simulink library "lib_converters"  (R2020b)
settings: Solver=VariableStepAuto  StartTime=0.0  StopTime=10.0  RelTol=1e-3
undefined symbols (not defined in the file): C_sc, DiscIntNeverNeededParam
libraries: powerlib x170, simulink x12, $bdroot x6, powerlib_meascontrol x3
(part 2 of 3)

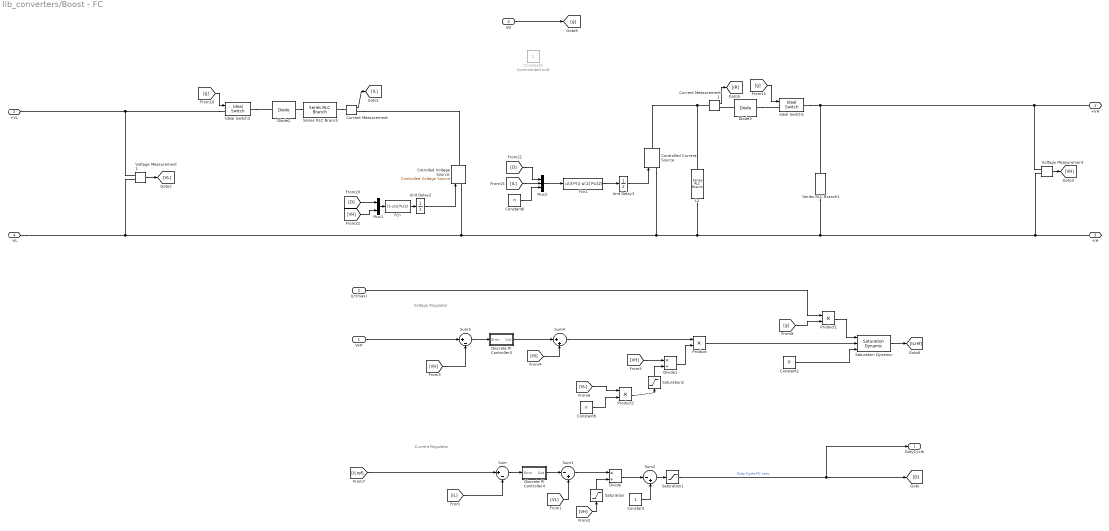
== system lib_converters/Boost - FC ==
  note: Current Regulator
  note: Voltage Regulator
  VH* : Inport
  IL*(max) : Inport  Port=2
  I/O : Inport  Port=3
  Constant : Constant
  Constant1 : Constant  Value=0
  Constant3 : Constant  Commented=on
  Constant6 : Constant  Value=n
  Constant8 : Constant  Value=n
  Controlled Current Source : powerlib/Electrical Sources/Controlled Current Source  Initialize=off  Source_Type=DC  Amplitude=0  Phase=0  Frequency=0  Measurements=None
  Cotrolled Voltage Source : powerlib/Electrical Sources/Controlled Voltage Source  Initialize=off  Source_Type=DC  Amplitude=0  Phase=0  Frequency=0  Measurements=None
  Current Measurement : powerlib/Measurements/Current Measurement  PhasorSimulation=off  OutputType=Complex  PSBequivalent=0
  Current Measurement1 : powerlib/Measurements/Current Measurement  PhasorSimulation=off  OutputType=Complex  PSBequivalent=0
  Diode2 : powerlib/Power Electronics/Diode  Ron=0.001  Lon=0  Vf=0  IC=0  UseSnubber=off  Rs=1e6  Cs=250e-9  Measurements=off
  Diode3 : powerlib/Power Electronics/Diode  Ron=0.001  Lon=0  Vf=0  IC=0  UseSnubber=off  Rs=1e6  Cs=250e-9  Measurements=off
  Discrete PI Controller3 : Subsystem  DialogController=POWERSYS.PowerSysDialog  mask(Discrete PI Controller){Kp=Kpv, Ki=Kiv, Par_Limits=[0.5 -0.5], Init=0, Ts=Tr}
      mask prompts: Kp "Proportional gain (Kp):"; Ki "Integral gain (Ki):"; Par_Limits "Output limits: [ Upper   Lower ]"; Init "Output initial value:"; Ts "Sample time:"
      mask help: This block implements a discrete PI controller.
      mask init:
      | UpperLimit=Par_Limits(1);
      | LowerLimit=Par_Limits(2);
      | power_initmask();
      mask Help: This block is part of a subset of blocks in the Extras library that does not have documentation associated with it, other than the block mask description.
      mask Display: disp('PI');
  Discrete PI Controller4 : Subsystem  DialogController=POWERSYS.PowerSysDialog  mask(Discrete PI Controller){Kp=Kpi/1000, Ki=Kii/1000, Par_Limits=[50 -50], Init=0, Ts=Ts}
      mask prompts: Kp "Proportional gain (Kp):"; Ki "Integral gain (Ki):"; Par_Limits "Output limits: [ Upper   Lower ]"; Init "Output initial value:"; Ts "Sample time:"
      mask help: This block implements a discrete PI controller.
      mask init:
      | UpperLimit=Par_Limits(1);
      | LowerLimit=Par_Limits(2);
      | power_initmask();
      mask Help: This block is part of a subset of blocks in the Extras library that does not have documentation associated with it, other than the block mask description.
      mask Display: disp('PI');
  Divide : Product  Inputs=*/  SampleTime=Ts
  Divide1 : Product  Inputs=*/  SampleTime=Ts
  Fcn : Fcn  Expr=(1-u(1))*u(2)
  Fcn1 : Fcn  Expr=u(3)*(1-u(1))*u(2)
  Ideal Switch1 : powerlib/Power Electronics/Ideal Switch  Ron=0.001  Lon=0  IC=0  Rs=1e5  Cs=inf  Measurements=off
  Ideal Switch3 : powerlib/Power Electronics/Ideal Switch  Ron=0.001  Lon=0  IC=0  Rs=1e5  Cs=inf  Measurements=off
  L2 : powerlib/Elements/Series RLC Branch  LConnTagsString=__new0  RConnTagsString=__new0  BranchType=C  Resistance=0.01  Inductance=100e-6  SetiL0=off  InitialCurrent=100  Capacitance=Co  Setx0=off  InitialVoltage=100  Measurements=None
  Mux1 : Mux  Inputs=2
  Mux2 : Mux  Inputs=3
  Product : Product  RndMeth=Zero
  Product1 : Product  RndMeth=Zero
  Product2 : Product  RndMeth=Zero
  Saturation : Saturate  UpperLimit=inf  LowerLimit=0.01  SampleTime=Ts
  Saturation Dynamic : simulink/Discontinuities/Saturation Dynamic  OutMin=[]  OutMax=[]  OutDataTypeStr=Inherit: Same as second input  OutDataType=fixdt(1, 16)  OutScaling=2^-10  DoSatur=off
  Saturation1 : Saturate  UpperLimit=1  LowerLimit=0  SampleTime=Ts
  Saturation2 : Saturate  UpperLimit=inf  LowerLimit=0.01  SampleTime=Ts
  Series RLC Branch : powerlib/Elements/Series RLC Branch  LConnTagsString=__new0  RConnTagsString=__new0  BranchType=L  Resistance=1  Inductance=L  SetiL0=off  InitialCurrent=1  Capacitance=1e-6  Setx0=off  InitialVoltage=0  Measurements=None
  Series RLC Branch1 : powerlib/Elements/Series RLC Branch  LConnTagsString=__new0  RConnTagsString=__new0  BranchType=R  Resistance=5e3  Inductance=1e-3  SetiL0=off  InitialCurrent=0  Capacitance=15  Setx0=on  InitialVoltage=270  Measurements=None
  Sum : Sum  Inputs=|+-
  Sum1 : Sum  Inputs=|-+
  Sum2 : Sum  Inputs=|-+
  Sum3 : Sum  Inputs=|+-
  Sum4 : Sum  Inputs=|++
  Unit Delay2 : UnitDelay  SampleTime=Ts  HasFrameUpgradeWarning=on
  Unit Delay3 : UnitDelay  SampleTime=Ts  HasFrameUpgradeWarning=on
  Voltage Measurement : powerlib/Measurements/Voltage Measurement  PhasorSimulation=off  OutputType=Complex  PSBequivalent=0
  Voltage Measurement1 : powerlib/Measurements/Voltage Measurement  PhasorSimulation=off  OutputType=Complex  PSBequivalent=0
  +VH : PMIOPort  Side=Right
  +VL : PMIOPort  Port=2  Side=Left
  -VH : PMIOPort  Port=3  Side=Right
  -VL : PMIOPort  Port=4  Side=Left
  DutyCycle : Outport
  wires:
  Product2/1 -> Saturation2/1
  Saturation1/1 -> [D], DutyCycle/1  "Duty Cycle FC conv"
  [IL] -> Mux2/2
  Sum3/1 -> Discrete PI Controller3/1(Error)
  [VH] -> Mux1/2
  Unit Delay3/1 -> Controlled Current Source/1
  Voltage Measurement/1 -> [VH]
  Discrete PI Controller3/1(Out) -> Sum4/1
  [D] -> Mux2/1
  Fcn1/1 -> Unit Delay3/1
  Fcn/1 -> Unit Delay2/1
  [D] -> Mux1/1
  Divide/1 -> Sum2/1
  Mux2/1 -> Fcn1/1
  Sum4/1 -> Product/1
  Constant8/1 -> Product2/2
  Constant6/1 -> Mux2/3
  IL*(max)/1 -> Product1/1
  Voltage Measurement1/1 -> [VL]
  Sum2/1 -> Saturation1/1
  Current Measurement1/1 -> [IR]
  [VH] -> Saturation/1
  Discrete PI Controller4/1(Out) -> Sum1/1
  [IL] -> Sum/2
  Sum/1 -> Discrete PI Controller4/1(Error)
  Product/1 -> Saturation Dynamic/2
  Constant/1 -> Sum2/2
  [VL] -> Product2/1
  Current Measurement/1 -> [IL]
  [VH] -> Sum3/2
  [VH] -> Divide1/1
  VH*/1 -> Sum3/1
  [IR] -> Sum4/2
  Mux1/1 -> Fcn/1
  Saturation/1 -> Divide/2
  Sum1/1 -> Divide/1
  [VL] -> Sum1/2
  Divide1/1 -> Product/2
  [ILref] -> Sum/1
  Constant1/1 -> Saturation Dynamic/3
  Saturation Dynamic/1 -> [ILref]
  [g] -> Ideal Switch3/1
  [g] -> Ideal Switch1/1
  Saturation2/1 -> Divide1/2
  [g] -> Product1/2
  Product1/1 -> Saturation Dynamic/1
  Unit Delay2/1 -> Cotrolled Voltage Source/1
  I/O/1 -> [g]
  connections:
  L2/LConn1 -- Controlled Current Source/RConn1 -- Current Measurement1/LConn1
  Ideal Switch3/LConn1 -- Voltage Measurement1/LConn1 -- +VL/RConn1
  Controlled Current Source/LConn1 -- L2/RConn1 -- -VH/RConn1 -- Voltage Measurement/LConn2 -- Series RLC Branch1/RConn1 -- Cotrolled Voltage Source/LConn1 -- Voltage Measurement1/LConn2 -- -VL/RConn1
  +VH/RConn1 -- Voltage Measurement/LConn1 -- Ideal Switch1/RConn1 -- Series RLC Branch1/LConn1
  Ideal Switch3/RConn1 -- Diode2/LConn1
  Diode2/RConn1 -- Series RLC Branch/LConn1
  Series RLC Branch/RConn1 -- Current Measurement/LConn1
  Current Measurement/RConn1 -- Cotrolled Voltage Source/RConn1
  Diode3/LConn1 -- Current Measurement1/RConn1
  Diode3/RConn1 -- Ideal Switch1/LConn1

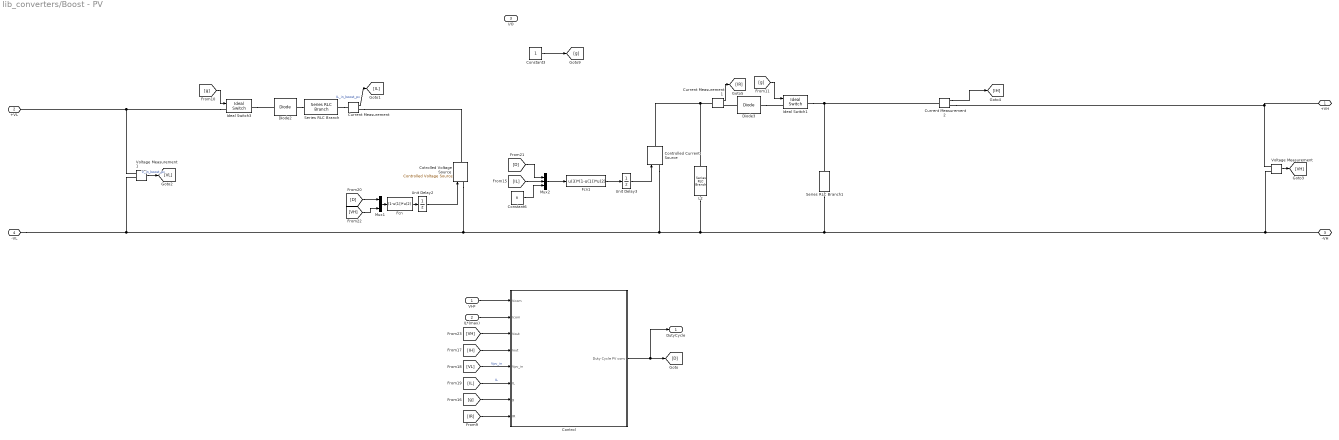
== system lib_converters/Boost - PV ==
  VH* : Inport
  IL*(max) : Inport  Port=2
  I/O : Inport  Port=3
  Constant3 : Constant
  Constant6 : Constant  Value=n
  Control : Subsystem  Variant=on  VariantControlMode=label  VariantControl=Choice  LabelModeActiveChoice=MPPT
  Controlled Current Source : powerlib/Electrical Sources/Controlled Current Source  Initialize=off  Source_Type=DC  Amplitude=0  Phase=0  Frequency=0  Measurements=None
  Cotrolled Voltage Source : powerlib/Electrical Sources/Controlled Voltage Source  Initialize=off  Source_Type=DC  Amplitude=0  Phase=0  Frequency=0  Measurements=None
  Current Measurement : powerlib/Measurements/Current Measurement  PhasorSimulation=off  OutputType=Complex  PSBequivalent=0
  Current Measurement1 : powerlib/Measurements/Current Measurement  PhasorSimulation=off  OutputType=Complex  PSBequivalent=0
  Current Measurement2 : powerlib/Measurements/Current Measurement  PhasorSimulation=off  OutputType=Complex  PSBequivalent=0
  Diode2 : powerlib/Power Electronics/Diode  Ron=0.001  Lon=0  Vf=0  IC=0  UseSnubber=off  Rs=1e6  Cs=250e-9  Measurements=off
  Diode3 : powerlib/Power Electronics/Diode  Ron=0.001  Lon=0  Vf=0  IC=0  UseSnubber=off  Rs=1e6  Cs=250e-9  Measurements=off
  Fcn : Fcn  Expr=(1-u(1))*u(2)
  Fcn1 : Fcn  Expr=u(3)*(1-u(1))*u(2)
  Ideal Switch1 : powerlib/Power Electronics/Ideal Switch  Ron=0.001  Lon=0  IC=0  Rs=1e5  Cs=inf  Measurements=off
  Ideal Switch3 : powerlib/Power Electronics/Ideal Switch  Ron=0.001  Lon=0  IC=0  Rs=1e5  Cs=inf  Measurements=off
  L2 : powerlib/Elements/Series RLC Branch  LConnTagsString=__new0  RConnTagsString=__new0  BranchType=C  Resistance=0.01  Inductance=100e-6  SetiL0=off  InitialCurrent=100  Capacitance=Co  Setx0=off  InitialVoltage=100  Measurements=None
  Mux1 : Mux  Inputs=2
  Mux2 : Mux  Inputs=3
  Series RLC Branch : powerlib/Elements/Series RLC Branch  LConnTagsString=__new0  RConnTagsString=__new0  BranchType=L  Resistance=1  Inductance=L  SetiL0=off  InitialCurrent=1  Capacitance=1e-6  Setx0=off  InitialVoltage=0  Measurements=None
  Series RLC Branch1 : powerlib/Elements/Series RLC Branch  LConnTagsString=__new0  RConnTagsString=__new0  BranchType=R  Resistance=5e3  Inductance=1e-3  SetiL0=off  InitialCurrent=0  Capacitance=15  Setx0=on  InitialVoltage=270  Measurements=None
  Unit Delay2 : UnitDelay  SampleTime=Ts  HasFrameUpgradeWarning=on
  Unit Delay3 : UnitDelay  SampleTime=Ts  HasFrameUpgradeWarning=on
  Voltage Measurement : powerlib/Measurements/Voltage Measurement  PhasorSimulation=off  OutputType=Complex  PSBequivalent=0
  Voltage Measurement1 : powerlib/Measurements/Voltage Measurement  PhasorSimulation=off  OutputType=Complex  PSBequivalent=0
  +VH : PMIOPort  Side=Right
  +VL : PMIOPort  Port=2  Side=Left
  -VH : PMIOPort  Port=3  Side=Right
  -VL : PMIOPort  Port=4  Side=Left
  DutyCycle : Outport
  wires:
  Constant3/1 -> [g]
  [IL] -> Mux2/2
  [VH] -> Mux1/2
  Unit Delay3/1 -> Controlled Current Source/1
  Voltage Measurement/1 -> [VH]
  [D] -> Mux2/1
  Fcn1/1 -> Unit Delay3/1
  Fcn/1 -> Unit Delay2/1
  [D] -> Mux1/1
  Mux2/1 -> Fcn1/1
  Constant6/1 -> Mux2/3
  IL*(max)/1 -> Control/2(Icom)
  Voltage Measurement1/1 -> [VL]  "V_in_boost_pv"
  Current Measurement1/1 -> [IR]
  Current Measurement/1 -> [IL]  "IL_in_boost_pv"
  VH*/1 -> Control/1(Vcom)
  Mux1/1 -> Fcn/1
  [g] -> Ideal Switch3/1
  [g] -> Ideal Switch1/1
  Unit Delay2/1 -> Cotrolled Voltage Source/1
  Current Measurement2/1 -> [IH]
  [VH] -> Control/3(Vout)
  [IH] -> Control/4(Iout)
  [VL] -> Control/5(Vpv_in)  "Vpv_in"
  [IL] -> Control/6(IL)  "IL"
  [g] -> Control/7(g)
  [IR] -> Control/8(IR)
  Control/1(Duty Cycle PV conv) -> DutyCycle/1, [D]
  connections:
  L2/LConn1 -- Controlled Current Source/RConn1 -- Current Measurement1/LConn1
  Ideal Switch3/LConn1 -- Voltage Measurement1/LConn1 -- +VL/RConn1
  Controlled Current Source/LConn1 -- L2/RConn1 -- -VH/RConn1 -- Voltage Measurement/LConn2 -- Series RLC Branch1/RConn1 -- Cotrolled Voltage Source/LConn1 -- Voltage Measurement1/LConn2 -- -VL/RConn1
  +VH/RConn1 -- Current Measurement2/RConn1 -- Voltage Measurement/LConn1
  Ideal Switch3/RConn1 -- Diode2/LConn1
  Diode2/RConn1 -- Series RLC Branch/LConn1
  Series RLC Branch/RConn1 -- Current Measurement/LConn1
  Current Measurement/RConn1 -- Cotrolled Voltage Source/RConn1
  Diode3/LConn1 -- Current Measurement1/RConn1
  Diode3/RConn1 -- Ideal Switch1/LConn1
  Ideal Switch1/RConn1 -- Current Measurement2/LConn1 -- Series RLC Branch1/LConn1

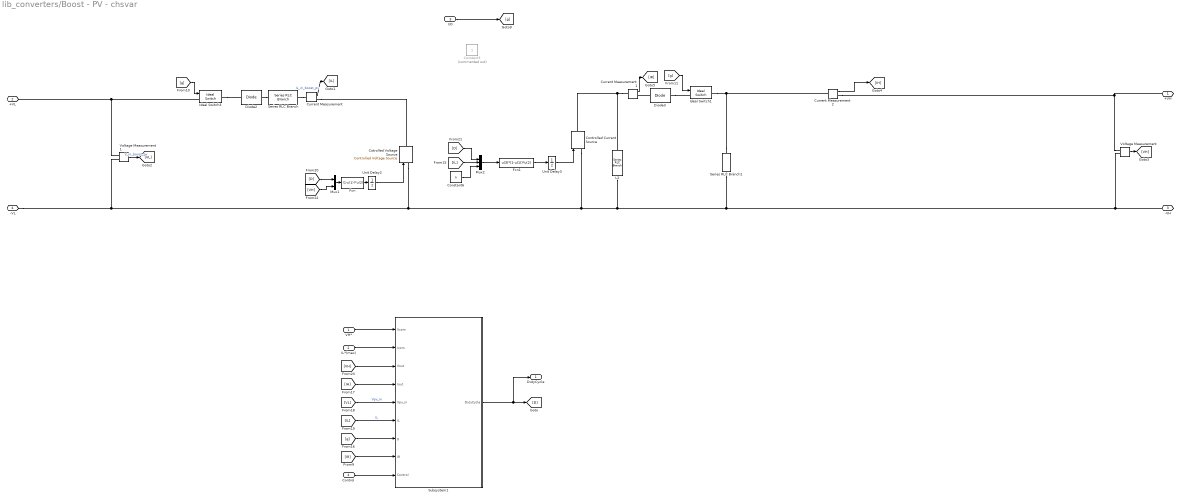
== system lib_converters/Boost - PV - chsvar ==
  VH* : Inport
  IL*(max) : Inport  Port=2
  I/O : Inport  Port=3
  Control : Inport  Port=4
  Constant3 : Constant  Commented=on
  Constant6 : Constant  Value=n
  Controlled Current Source : powerlib/Electrical Sources/Controlled Current Source  Initialize=off  Source_Type=DC  Amplitude=0  Phase=0  Frequency=0  Measurements=None
  Cotrolled Voltage Source : powerlib/Electrical Sources/Controlled Voltage Source  Initialize=off  Source_Type=DC  Amplitude=0  Phase=0  Frequency=0  Measurements=None
  Current Measurement : powerlib/Measurements/Current Measurement  PhasorSimulation=off  OutputType=Complex  PSBequivalent=0
  Current Measurement1 : powerlib/Measurements/Current Measurement  PhasorSimulation=off  OutputType=Complex  PSBequivalent=0
  Current Measurement2 : powerlib/Measurements/Current Measurement  PhasorSimulation=off  OutputType=Complex  PSBequivalent=0
  Diode2 : powerlib/Power Electronics/Diode  Ron=0.001  Lon=0  Vf=0  IC=0  UseSnubber=off  Rs=1e6  Cs=250e-9  Measurements=off
  Diode3 : powerlib/Power Electronics/Diode  Ron=0.001  Lon=0  Vf=0  IC=0  UseSnubber=off  Rs=1e6  Cs=250e-9  Measurements=off
  Fcn : Fcn  Expr=(1-u(1))*u(2)
  Fcn1 : Fcn  Expr=u(3)*(1-u(1))*u(2)
  Ideal Switch1 : powerlib/Power Electronics/Ideal Switch  Ron=0.001  Lon=0  IC=0  Rs=1e5  Cs=inf  Measurements=off
  Ideal Switch3 : powerlib/Power Electronics/Ideal Switch  Ron=0.001  Lon=0  IC=0  Rs=1e5  Cs=inf  Measurements=off
  L2 : powerlib/Elements/Series RLC Branch  LConnTagsString=__new0  RConnTagsString=__new0  BranchType=C  Resistance=0.01  Inductance=100e-6  SetiL0=off  InitialCurrent=100  Capacitance=Co  Setx0=off  InitialVoltage=100  Measurements=None
  Mux1 : Mux  Inputs=2
  Mux2 : Mux  Inputs=3
  Series RLC Branch : powerlib/Elements/Series RLC Branch  LConnTagsString=__new0  RConnTagsString=__new0  BranchType=L  Resistance=1  Inductance=L  SetiL0=off  InitialCurrent=1  Capacitance=1e-6  Setx0=off  InitialVoltage=0  Measurements=None
  Series RLC Branch1 : powerlib/Elements/Series RLC Branch  LConnTagsString=__new0  RConnTagsString=__new0  BranchType=R  Resistance=5e3  Inductance=1e-3  SetiL0=off  InitialCurrent=0  Capacitance=15  Setx0=on  InitialVoltage=270  Measurements=None
  Subsystem1 : Subsystem
  Unit Delay2 : UnitDelay  SampleTime=Ts  HasFrameUpgradeWarning=on
  Unit Delay3 : UnitDelay  SampleTime=Ts  HasFrameUpgradeWarning=on
  Voltage Measurement : powerlib/Measurements/Voltage Measurement  PhasorSimulation=off  OutputType=Complex  PSBequivalent=0
  Voltage Measurement1 : powerlib/Measurements/Voltage Measurement  PhasorSimulation=off  OutputType=Complex  PSBequivalent=0
  +VH : PMIOPort  Side=Right
  +VL : PMIOPort  Port=2  Side=Left
  -VH : PMIOPort  Port=3  Side=Right
  -VL : PMIOPort  Port=4  Side=Left
  DutyCycle : Outport
  wires:
  Subsystem1/1(DutyCycle) -> [D], DutyCycle/1
  [IR] -> Subsystem1/8(IR)
  [g] -> Subsystem1/7(g)
  [IL] -> Subsystem1/6(IL)  "IL"
  [VL] -> Subsystem1/5(Vpv_in)  "Vpv_in"
  [IH] -> Subsystem1/4(Iout)
  [VH] -> Subsystem1/3(Vout)
  Current Measurement2/1 -> [IH]
  Unit Delay2/1 -> Cotrolled Voltage Source/1
  [g] -> Ideal Switch1/1
  [g] -> Ideal Switch3/1
  Mux1/1 -> Fcn/1
  VH*/1 -> Subsystem1/1(Vcom)
  Current Measurement/1 -> [IL]  "IL_in_boost_pv"
  Current Measurement1/1 -> [IR]
  Voltage Measurement1/1 -> [VL]  "V_in_boost_pv"
  IL*(max)/1 -> Subsystem1/2(Icom)
  Constant6/1 -> Mux2/3
  Mux2/1 -> Fcn1/1
  [D] -> Mux1/1
  Fcn/1 -> Unit Delay2/1
  Fcn1/1 -> Unit Delay3/1
  [D] -> Mux2/1
  Voltage Measurement/1 -> [VH]
  Unit Delay3/1 -> Controlled Current Source/1
  [VH] -> Mux1/2
  [IL] -> Mux2/2
  Control/1 -> Subsystem1/9(Control)
  I/O/1 -> [g]
  connections:
  Series RLC Branch1/LConn1 -- Current Measurement2/LConn1 -- Ideal Switch1/RConn1
  Diode3/RConn1 -- Ideal Switch1/LConn1
  Diode3/LConn1 -- Current Measurement1/RConn1
  Current Measurement/RConn1 -- Cotrolled Voltage Source/RConn1
  Series RLC Branch/RConn1 -- Current Measurement/LConn1
  Diode2/RConn1 -- Series RLC Branch/LConn1
  Ideal Switch3/RConn1 -- Diode2/LConn1
  Voltage Measurement/LConn1 -- Current Measurement2/RConn1 -- +VH/RConn1
  -VL/RConn1 -- Voltage Measurement1/LConn2 -- Cotrolled Voltage Source/LConn1 -- Series RLC Branch1/RConn1 -- Voltage Measurement/LConn2 -- -VH/RConn1 -- L2/RConn1 -- Controlled Current Source/LConn1
  +VL/RConn1 -- Voltage Measurement1/LConn1 -- Ideal Switch3/LConn1
  Current Measurement1/LConn1 -- Controlled Current Source/RConn1 -- L2/LConn1

== system lib_converters/Boost - PV - fast ==
  I/O : Inport
  Constant6 : Constant  Value=n
  Controlled Current Source : powerlib/Electrical Sources/Controlled Current Source  Initialize=off  Source_Type=DC  Amplitude=0  Phase=0  Frequency=0  Measurements=None
  Cotrolled Voltage Source : powerlib/Electrical Sources/Controlled Voltage Source  Initialize=off  Source_Type=DC  Amplitude=0  Phase=0  Frequency=0  Measurements=None
  Current Measurement : powerlib/Measurements/Current Measurement  PhasorSimulation=off  OutputType=Complex  PSBequivalent=0
  Current Measurement1 : powerlib/Measurements/Current Measurement  PhasorSimulation=off  OutputType=Complex  PSBequivalent=0
  Current Measurement2 : powerlib/Measurements/Current Measurement  PhasorSimulation=off  OutputType=Complex  PSBequivalent=0
  Diode2 : powerlib/Power Electronics/Diode  Ron=0.001  Lon=0  Vf=0  IC=0  UseSnubber=off  Rs=1e6  Cs=250e-9  Measurements=off
  Diode3 : powerlib/Power Electronics/Diode  Ron=0.001  Lon=0  Vf=0  IC=0  UseSnubber=off  Rs=1e6  Cs=250e-9  Measurements=off
  Fcn : Fcn  Expr=(1-u(1))*u(2)
  Fcn1 : Fcn  Expr=u(3)*(1-u(1))*u(2)
  Ideal Switch1 : powerlib/Power Electronics/Ideal Switch  Ron=0.001  Lon=0  IC=0  Rs=1e5  Cs=inf  Measurements=off
  Ideal Switch3 : powerlib/Power Electronics/Ideal Switch  Ron=0.001  Lon=0  IC=0  Rs=1e5  Cs=inf  Measurements=off
  L2 : powerlib/Elements/Series RLC Branch  LConnTagsString=__new0  RConnTagsString=__new0  BranchType=C  Resistance=0.01  Inductance=100e-6  SetiL0=off  InitialCurrent=100  Capacitance=Co  Setx0=off  InitialVoltage=100  Measurements=None
  MPPT : MATLAB Function  TreatAsAtomicUnit=on
  Mux1 : Mux  Inputs=2
  Mux2 : Mux  Inputs=3
  Saturation1 : Saturate  UpperLimit=1  LowerLimit=0  SampleTime=Ts
  Series RLC Branch : powerlib/Elements/Series RLC Branch  LConnTagsString=__new0  RConnTagsString=__new0  BranchType=L  Resistance=1  Inductance=L  SetiL0=off  InitialCurrent=1  Capacitance=1e-6  Setx0=off  InitialVoltage=0  Measurements=None
  Series RLC Branch1 : powerlib/Elements/Series RLC Branch  LConnTagsString=__new0  RConnTagsString=__new0  BranchType=R  Resistance=5e3  Inductance=1e-3  SetiL0=off  InitialCurrent=0  Capacitance=15  Setx0=on  InitialVoltage=270  Measurements=None
  Unit Delay1 : UnitDelay  SampleTime=Ts*10  HasFrameUpgradeWarning=on
  Unit Delay2 : UnitDelay  SampleTime=Ts  HasFrameUpgradeWarning=on
  Unit Delay3 : UnitDelay  SampleTime=Ts  HasFrameUpgradeWarning=on
  Voltage Measurement : powerlib/Measurements/Voltage Measurement  PhasorSimulation=off  OutputType=Complex  PSBequivalent=0
  Voltage Measurement1 : powerlib/Measurements/Voltage Measurement  PhasorSimulation=off  OutputType=Complex  PSBequivalent=0
  +VH : PMIOPort  Side=Right
  +VL : PMIOPort  Port=2  Side=Left
  -VH : PMIOPort  Port=3  Side=Right
  -VL : PMIOPort  Port=4  Side=Left
  wires:
  [IL] -> MPPT/2(I_L)  "IL"
  [VL] -> MPPT/1(Vpv_in)  "Vpv_in"
  Current Measurement2/1 -> [IH]
  Unit Delay2/1 -> Cotrolled Voltage Source/1
  [g] -> Ideal Switch1/1
  [g] -> Ideal Switch3/1
  Mux1/1 -> Fcn/1
  Current Measurement/1 -> [IL]  "IL_in_boost_pv"
  Current Measurement1/1 -> [IR]
  Voltage Measurement1/1 -> [VL]  "V_in_boost_pv"
  Constant6/1 -> Mux2/3
  Mux2/1 -> Fcn1/1
  [D] -> Mux1/1
  Fcn/1 -> Unit Delay2/1
  Fcn1/1 -> Unit Delay3/1
  [D] -> Mux2/1
  Voltage Measurement/1 -> [VH]
  Unit Delay3/1 -> Controlled Current Source/1
  [VH] -> Mux1/2
  [IL] -> Mux2/2
  I/O/1 -> [g]
  Unit Delay1/1 -> Saturation1/1
  MPPT/1(D) -> Unit Delay1/1
  Saturation1/1 -> [D]  "Duty Cycle PV conv"
  connections:
  Series RLC Branch1/LConn1 -- Current Measurement2/LConn1 -- Ideal Switch1/RConn1
  Diode3/RConn1 -- Ideal Switch1/LConn1
  Diode3/LConn1 -- Current Measurement1/RConn1
  Current Measurement/RConn1 -- Cotrolled Voltage Source/RConn1
  Series RLC Branch/RConn1 -- Current Measurement/LConn1
  Diode2/RConn1 -- Series RLC Branch/LConn1
  Ideal Switch3/RConn1 -- Diode2/LConn1
  Voltage Measurement/LConn1 -- Current Measurement2/RConn1 -- +VH/RConn1
  -VL/RConn1 -- Voltage Measurement1/LConn2 -- Cotrolled Voltage Source/LConn1 -- Series RLC Branch1/RConn1 -- Voltage Measurement/LConn2 -- -VH/RConn1 -- L2/RConn1 -- Controlled Current Source/LConn1
  +VL/RConn1 -- Voltage Measurement1/LConn1 -- Ideal Switch3/LConn1
  Current Measurement1/LConn1 -- Controlled Current Source/RConn1 -- L2/LConn1

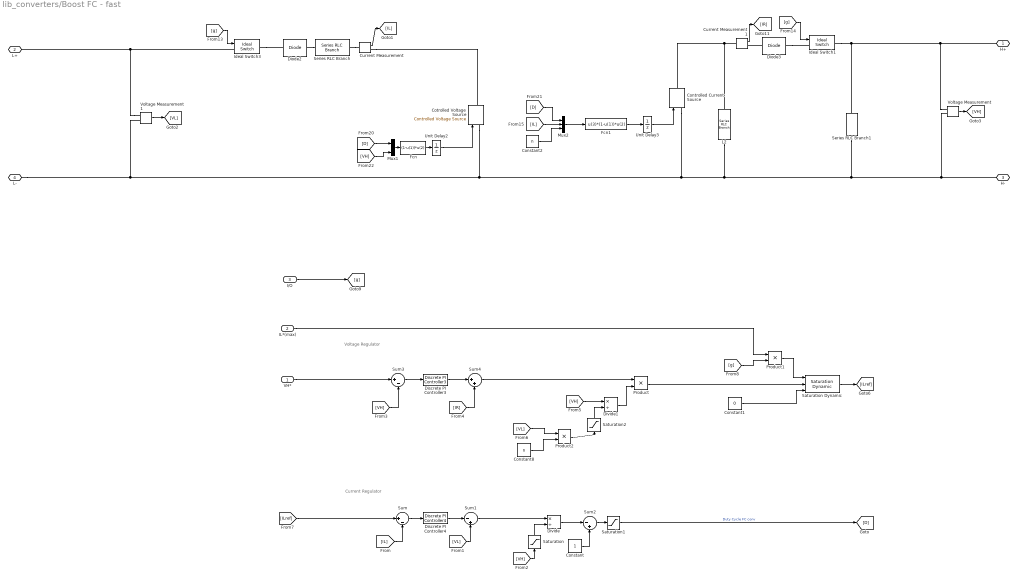
== system lib_converters/Boost FC - fast ==
  note: Voltage Regulator
  note: Current Regulator
  VH* : Inport
  IL*(max) : Inport  Port=2
  I/O : Inport  Port=3
  Constant : Constant
  Constant1 : Constant  Value=0
  Constant2 : Constant  Value=n
  Constant8 : Constant  Value=n
  Controlled Current Source : powerlib/Electrical Sources/Controlled Current Source  Initialize=off  Source_Type=DC  Amplitude=0  Phase=0  Frequency=0  Measurements=None
  Cotrolled Voltage Source : powerlib/Electrical Sources/Controlled Voltage Source  Initialize=off  Source_Type=DC  Amplitude=0  Phase=0  Frequency=0  Measurements=None
  Current Measurement : powerlib/Measurements/Current Measurement  PhasorSimulation=off  OutputType=Complex  PSBequivalent=0
  Current Measurement1 : powerlib/Measurements/Current Measurement  PhasorSimulation=off  OutputType=Complex  PSBequivalent=0
  Diode2 : powerlib/Power Electronics/Diode  Ron=0.001  Lon=0  Vf=0  IC=0  UseSnubber=off  Rs=1e6  Cs=250e-9  Measurements=off
  Diode3 : powerlib/Power Electronics/Diode  Ron=0.001  Lon=0  Vf=0  IC=0  UseSnubber=off  Rs=1e6  Cs=250e-9  Measurements=off
  Discrete PI Controller3 : $bdroot/Boost - FC/Discrete PI Controller3  Kp=Kpv  Ki=Kiv  Par_Limits=[0.5 -0.5]  Init=0  Ts=Ts
  Discrete PI Controller4 : $bdroot/Boost - FC/Discrete PI Controller4  Kp=Kpi/1000  Ki=Kii/1000  Par_Limits=[50 -50]  Init=0  Ts=Ts
  Divide : Product  Inputs=*/  SampleTime=Ts
  Divide1 : Product  Inputs=*/  SampleTime=Ts
  Fcn : Fcn  Expr=(1-u(1))*u(2)
  Fcn1 : Fcn  Expr=u(3)*(1-u(1))*u(2)
  Ideal Switch1 : powerlib/Power Electronics/Ideal Switch  Ron=0.001  Lon=0  IC=0  Rs=1e5  Cs=inf  Measurements=off
  Ideal Switch3 : powerlib/Power Electronics/Ideal Switch  Ron=0.001  Lon=0  IC=0  Rs=1e5  Cs=inf  Measurements=off
  L2 : powerlib/Elements/Series RLC Branch  LConnTagsString=__new0  RConnTagsString=__new0  BranchType=C  Resistance=0.01  Inductance=100e-6  SetiL0=off  InitialCurrent=100  Capacitance=Co  Setx0=off  InitialVoltage=100  Measurements=None
  Mux1 : Mux  Inputs=2
  Mux2 : Mux  Inputs=3
  Product : Product  RndMeth=Zero
  Product1 : Product  RndMeth=Zero
  Product2 : Product  RndMeth=Zero
  Saturation : Saturate  UpperLimit=inf  LowerLimit=0.01  SampleTime=Ts
  Saturation Dynamic : simulink/Discontinuities/Saturation Dynamic  OutMin=[]  OutMax=[]  OutDataTypeStr=Inherit: Same as second input  OutDataType=fixdt(1, 16)  OutScaling=2^-10  DoSatur=off
  Saturation1 : Saturate  UpperLimit=1  LowerLimit=0  SampleTime=Ts
  Saturation2 : Saturate  UpperLimit=inf  LowerLimit=0.01  SampleTime=Ts
  Series RLC Branch : powerlib/Elements/Series RLC Branch  LConnTagsString=__new0  RConnTagsString=__new0  BranchType=L  Resistance=1  Inductance=L  SetiL0=off  InitialCurrent=1  Capacitance=1e-6  Setx0=off  InitialVoltage=0  Measurements=None
  Series RLC Branch1 : powerlib/Elements/Series RLC Branch  LConnTagsString=__new0  RConnTagsString=__new0  BranchType=R  Resistance=5e3  Inductance=1e-3  SetiL0=off  InitialCurrent=0  Capacitance=15  Setx0=on  InitialVoltage=270  Measurements=None
  Sum : Sum  Inputs=|+-
  Sum1 : Sum  Inputs=|-+
  Sum2 : Sum  Inputs=|-+
  Sum3 : Sum  Inputs=|+-
  Sum4 : Sum  Inputs=|++
  Unit Delay2 : UnitDelay  SampleTime=Ts  HasFrameUpgradeWarning=on
  Unit Delay3 : UnitDelay  SampleTime=Ts  HasFrameUpgradeWarning=on
  Voltage Measurement : powerlib/Measurements/Voltage Measurement  PhasorSimulation=off  OutputType=Complex  PSBequivalent=0
  Voltage Measurement1 : powerlib/Measurements/Voltage Measurement  PhasorSimulation=off  OutputType=Complex  PSBequivalent=0
  H+ : PMIOPort  Side=Right
  L+ : PMIOPort  Port=2  Side=Left
  H- : PMIOPort  Port=3  Side=Right
  L- : PMIOPort  Port=4  Side=Left
  wires:
  IL*(max)/1 -> Product1/1
  Divide1/1 -> Product/2
  [ILref] -> Sum/1
  Sum1/1 -> Divide/1
  [VH] -> Divide1/1
  [VL] -> Sum1/2
  [IR] -> Sum4/2
  Constant/1 -> Sum2/2
  Product/1 -> Saturation Dynamic/2
  [IL] -> Sum/2
  Discrete PI Controller4/1 -> Sum1/1
  Divide/1 -> Sum2/1
  Saturation1/1 -> [D]  "Duty Cycle FC conv"
  Constant8/1 -> Product2/2
  Sum3/1 -> Discrete PI Controller3/1
  VH*/1 -> Sum3/1
  I/O/1 -> [g]
  Saturation2/1 -> Divide1/2
  Constant1/1 -> Saturation Dynamic/3
  Sum2/1 -> Saturation1/1
  [VL] -> Product2/1
  [g] -> Product1/2
  Saturation Dynamic/1 -> [ILref]
  Saturation/1 -> Divide/2
  [VH] -> Saturation/1
  Discrete PI Controller3/1 -> Sum4/1
  [VH] -> Sum3/2
  Product1/1 -> Saturation Dynamic/1
  Product2/1 -> Saturation2/1
  Sum4/1 -> Product/1
  Sum/1 -> Discrete PI Controller4/1
  [g] -> Ideal Switch1/1
  Voltage Measurement1/1 -> [VL]
  Current Measurement/1 -> [IL]
  Fcn/1 -> Unit Delay2/1
  [D] -> Mux2/1
  Unit Delay2/1 -> Cotrolled Voltage Source/1
  Mux1/1 -> Fcn/1
  Voltage Measurement/1 -> [VH]
  [VH] -> Mux1/2
  Current Measurement1/1 -> [IR]
  Mux2/1 -> Fcn1/1
  Unit Delay3/1 -> Controlled Current Source/1
  [D] -> Mux1/1
  Fcn1/1 -> Unit Delay3/1
  Constant2/1 -> Mux2/3
  [g] -> Ideal Switch3/1
  [IL] -> Mux2/2
  connections:
  Voltage Measurement/LConn1 -- H+/RConn1 -- Series RLC Branch1/LConn1 -- Ideal Switch1/RConn1
  Voltage Measurement/LConn2 -- Series RLC Branch1/RConn1 -- Controlled Current Source/LConn1 -- Cotrolled Voltage Source/LConn1 -- Voltage Measurement1/LConn2 -- L-/RConn1 -- L2/RConn1 -- H-/RConn1
  Controlled Current Source/RConn1 -- Current Measurement1/LConn1 -- L2/LConn1
  Voltage Measurement1/LConn1 -- L+/RConn1 -- Ideal Switch3/LConn1
  Diode3/LConn1 -- Current Measurement1/RConn1
  Ideal Switch3/RConn1 -- Diode2/LConn1
  Diode3/RConn1 -- Ideal Switch1/LConn1
  Series RLC Branch/RConn1 -- Current Measurement/LConn1
  Current Measurement/RConn1 -- Cotrolled Voltage Source/RConn1
  Diode2/RConn1 -- Series RLC Branch/LConn1

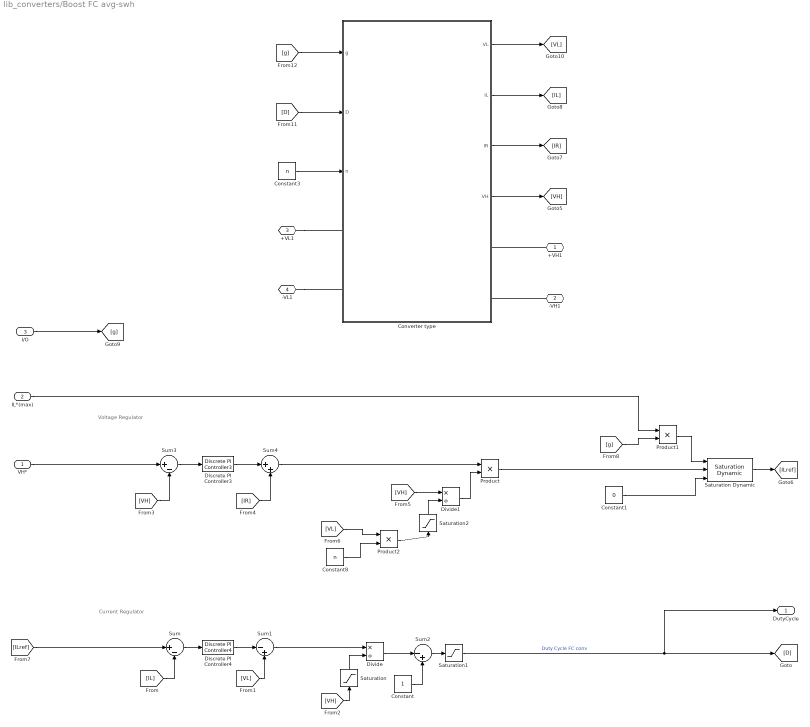
== system lib_converters/Boost FC avg-swh ==
  note: Voltage Regulator
  note: Current Regulator
  VH* : Inport
  IL*(max) : Inport  Port=2
  I/O : Inport  Port=3
  Constant : Constant
  Constant1 : Constant  Value=0
  Constant3 : Constant  Value=n
  Constant8 : Constant  Value=n
  Converter type : Subsystem  Variant=on  VariantControlMode=label  VariantControl=Choice  LabelModeActiveChoice=Choice
  Discrete PI Controller3 : $bdroot/Boost - FC/Discrete PI Controller3  Kp=Kpv  Ki=Kiv  Par_Limits=[0.5 -0.5]  Init=0  Ts=Ts
  Discrete PI Controller4 : $bdroot/Boost - FC/Discrete PI Controller4  Kp=Kpi/1000  Ki=Kii/1000  Par_Limits=[50 -50]  Init=0  Ts=Ts
  Divide : Product  Inputs=*/  SampleTime=Ts
  Divide1 : Product  Inputs=*/  SampleTime=Ts
  Product : Product  RndMeth=Zero
  Product1 : Product  RndMeth=Zero
  Product2 : Product  RndMeth=Zero
  Saturation : Saturate  UpperLimit=inf  LowerLimit=0.01  SampleTime=Ts
  Saturation Dynamic : simulink/Discontinuities/Saturation Dynamic  OutMin=[]  OutMax=[]  OutDataTypeStr=Inherit: Same as second input  OutDataType=fixdt(1, 16)  OutScaling=2^-10  DoSatur=off
  Saturation1 : Saturate  UpperLimit=1  LowerLimit=0  SampleTime=Ts
  Saturation2 : Saturate  UpperLimit=inf  LowerLimit=0.01  SampleTime=Ts
  Sum : Sum  Inputs=|+-
  Sum1 : Sum  Inputs=|-+
  Sum2 : Sum  Inputs=|-+
  Sum3 : Sum  Inputs=|+-
  Sum4 : Sum  Inputs=|++
  +VH1 : PMIOPort  Side=Right
  -VH1 : PMIOPort  Port=2  Side=Right
  +VL1 : PMIOPort  Port=3  Side=Left
  -VL1 : PMIOPort  Port=4  Side=Left
  DutyCycle : Outport
  wires:
  IL*(max)/1 -> Product1/1
  Divide1/1 -> Product/2
  [ILref] -> Sum/1
  Sum1/1 -> Divide/1
  [VH] -> Divide1/1
  [VL] -> Sum1/2
  [IR] -> Sum4/2
  Constant/1 -> Sum2/2
  Product/1 -> Saturation Dynamic/2
  [IL] -> Sum/2
  Discrete PI Controller4/1 -> Sum1/1
  Divide/1 -> Sum2/1
  Saturation1/1 -> [D], DutyCycle/1  "Duty Cycle FC conv"
  Constant8/1 -> Product2/2
  Sum3/1 -> Discrete PI Controller3/1
  VH*/1 -> Sum3/1
  I/O/1 -> [g]
  Saturation2/1 -> Divide1/2
  Constant1/1 -> Saturation Dynamic/3
  Sum2/1 -> Saturation1/1
  [VL] -> Product2/1
  [g] -> Product1/2
  Saturation Dynamic/1 -> [ILref]
  Saturation/1 -> Divide/2
  [VH] -> Saturation/1
  Discrete PI Controller3/1 -> Sum4/1
  [VH] -> Sum3/2
  Product1/1 -> Saturation Dynamic/1
  Product2/1 -> Saturation2/1
  Sum4/1 -> Product/1
  Sum/1 -> Discrete PI Controller4/1
  Converter type/4(VH) -> [VH]
  Converter type/3(IR) -> [IR]
  Converter type/2(IL) -> [IL]
  Converter type/1(VL) -> [VL]
  [g] -> Converter type/1(g)
  [D] -> Converter type/2(D)
  Constant3/1 -> Converter type/3(n)
  connections:
  -VH1/RConn1 -- Converter type/RConn2
  +VH1/RConn1 -- Converter type/RConn1
  +VL1/RConn1 -- Converter type/LConn1
  -VL1/RConn1 -- Converter type/LConn2

== system lib_converters/Boost FC swh ==
  note: Current Regulator
  note: Voltage Regulator
  VH* : Inport
  IL*(max) : Inport  Port=2
  I/O : Inport  Port=3
  Constant : Constant
  Constant1 : Constant  Value=0
  Constant3 : Constant  Value=n
  Constant8 : Constant  Value=n
  Converter type : Subsystem  Variant=on  VariantControlMode=label  VariantControl=Choice  LabelModeActiveChoice=Choice_1
  Discrete PI Controller3 : $bdroot/Boost - FC/Discrete PI Controller3  Kp=Kpv  Ki=Kiv  Par_Limits=[0.5 -0.5]  Init=0  Ts=Tr
  Discrete PI Controller4 : $bdroot/Boost - FC/Discrete PI Controller4  Kp=Kpi/1000  Ki=Kii/1000  Par_Limits=[50 -50]  Init=0  Ts=Ts
  Divide : Product  Inputs=*/  SampleTime=Ts
  Divide1 : Product  Inputs=*/  SampleTime=Ts
  Product : Product  RndMeth=Zero
  Product1 : Product  RndMeth=Zero
  Product2 : Product  RndMeth=Zero
  Saturation : Saturate  UpperLimit=inf  LowerLimit=0.01  SampleTime=Ts
  Saturation Dynamic : simulink/Discontinuities/Saturation Dynamic  OutMin=[]  OutMax=[]  OutDataTypeStr=Inherit: Same as second input  OutDataType=fixdt(1, 16)  OutScaling=2^-10  DoSatur=off
  Saturation1 : Saturate  UpperLimit=1  LowerLimit=0  SampleTime=Ts
  Saturation2 : Saturate  UpperLimit=inf  LowerLimit=0.01  SampleTime=Ts
  Sum : Sum  Inputs=|+-
  Sum1 : Sum  Inputs=|-+
  Sum2 : Sum  Inputs=|-+
  Sum3 : Sum  Inputs=|+-
  Sum4 : Sum  Inputs=|++
  +VH1 : PMIOPort  Side=Right
  -VH1 : PMIOPort  Port=2  Side=Right
  +VL1 : PMIOPort  Port=3  Side=Left
  -VL1 : PMIOPort  Port=4  Side=Left
  DutyCycle : Outport
  wires:
  Constant3/1 -> Converter type/3(n)
  [D] -> Converter type/2(D)
  [g] -> Converter type/1(g)
  Converter type/1(VL) -> [VL]
  Converter type/2(IL) -> [IL]
  Converter type/3(IR) -> [IR]
  Converter type/4(VH) -> [VH]
  Sum/1 -> Discrete PI Controller4/1
  Sum4/1 -> Product/1
  Product2/1 -> Saturation2/1
  Product1/1 -> Saturation Dynamic/1
  [VH] -> Sum3/2
  Discrete PI Controller3/1 -> Sum4/1
  [VH] -> Saturation/1
  Saturation/1 -> Divide/2
  Saturation Dynamic/1 -> [ILref]
  [g] -> Product1/2
  [VL] -> Product2/1
  Sum2/1 -> Saturation1/1
  Constant1/1 -> Saturation Dynamic/3
  Saturation2/1 -> Divide1/2
  I/O/1 -> [g]
  VH*/1 -> Sum3/1
  Sum3/1 -> Discrete PI Controller3/1
  Constant8/1 -> Product2/2
  Saturation1/1 -> DutyCycle/1, [D]  "Duty Cycle FC conv"
  Divide/1 -> Sum2/1
  Discrete PI Controller4/1 -> Sum1/1
  [IL] -> Sum/2
  Product/1 -> Saturation Dynamic/2
  Constant/1 -> Sum2/2
  [IR] -> Sum4/2
  [VL] -> Sum1/2
  [VH] -> Divide1/1
  Sum1/1 -> Divide/1
  [ILref] -> Sum/1
  Divide1/1 -> Product/2
  IL*(max)/1 -> Product1/1
  connections:
  -VL1/RConn1 -- Converter type/LConn2
  +VL1/RConn1 -- Converter type/LConn1
  +VH1/RConn1 -- Converter type/RConn1
  -VH1/RConn1 -- Converter type/RConn2

== system lib_converters/Bidirectional BOOST//BUCK - Batt/Discrete PI Controller1 ==
  note: Pierre Giroux, Gilbert Sybille
      | Power System Simulation Laboratory
      | IREQ, Hydro-Quebc
  note: Discrete PID Controller
  Error : Inport  SampleTime=Ts
  Discrete-Time Integrator : DiscreteIntegrator  InitialCondition=Init  SampleTime=Ts  LimitOutput=on  UpperSaturationLimit=UpperLimit  LowerSaturationLimit=LowerLimit  ICPrevOutput=DiscIntNeverNeededParam  ICPrevScaledInput=DiscIntNeverNeededParam
  Kp4 : Gain  Gain=Kp  SaturateOnIntegerOverflow=on  SampleTime=Ts  OutDataTypeStr=Inherit: Same as input  ParamDataTypeStr=Inherit: Same as input
  Kp5 : Gain  Gain=Ki  SaturateOnIntegerOverflow=on  SampleTime=Ts  OutDataTypeStr=Inherit: Same as input  ParamDataTypeStr=Inherit: Same as input
  Saturation2 : Saturate  UpperLimit=UpperLimit  LowerLimit=LowerLimit  SampleTime=Ts
  Sum6 : Sum  InputSameDT=on  SaturateOnIntegerOverflow=on  SampleTime=Ts  OutDataTypeStr=Inherit: Same as first input
  Zero-Order Hold : ZeroOrderHold  SampleTime=Ts
  Out : Outport  SampleTime=Ts  InitialOutput=0  VectorParamsAs1DForOutWhenUnconnected=off
  wires:
  Error/1 -> Kp4/1, Kp5/1
  Sum6/1 -> Saturation2/1
  Kp5/1 -> Discrete-Time Integrator/1
  Kp4/1 -> Zero-Order Hold/1
  Discrete-Time Integrator/1 -> Sum6/2
  Saturation2/1 -> Out/1
  Zero-Order Hold/1 -> Sum6/1

== system lib_converters/Bidirectional BOOST//BUCK - Batt/Discrete PI Controller2 ==
  note: Discrete PID Controller
  note: Pierre Giroux, Gilbert Sybille
      | Power System Simulation Laboratory
      | IREQ, Hydro-Quebc
  Error : Inport  SampleTime=Ts
  Discrete-Time Integrator : DiscreteIntegrator  InitialCondition=Init  SampleTime=Ts  LimitOutput=on  UpperSaturationLimit=UpperLimit  LowerSaturationLimit=LowerLimit  ICPrevOutput=DiscIntNeverNeededParam  ICPrevScaledInput=DiscIntNeverNeededParam
  Kp4 : Gain  Gain=Kp  SaturateOnIntegerOverflow=on  SampleTime=Ts  OutDataTypeStr=Inherit: Same as input  ParamDataTypeStr=Inherit: Same as input
  Kp5 : Gain  Gain=Ki  SaturateOnIntegerOverflow=on  SampleTime=Ts  OutDataTypeStr=Inherit: Same as input  ParamDataTypeStr=Inherit: Same as input
  Saturation2 : Saturate  UpperLimit=UpperLimit  LowerLimit=LowerLimit  SampleTime=Ts
  Sum6 : Sum  InputSameDT=on  SaturateOnIntegerOverflow=on  SampleTime=Ts  OutDataTypeStr=Inherit: Same as first input
  Zero-Order Hold : ZeroOrderHold  SampleTime=Ts
  Out : Outport  SampleTime=Ts  InitialOutput=0  VectorParamsAs1DForOutWhenUnconnected=off
  wires:
  Zero-Order Hold/1 -> Sum6/1
  Saturation2/1 -> Out/1
  Discrete-Time Integrator/1 -> Sum6/2
  Kp4/1 -> Zero-Order Hold/1
  Kp5/1 -> Discrete-Time Integrator/1
  Sum6/1 -> Saturation2/1
  Error/1 -> Kp5/1, Kp4/1

== system lib_converters/Bidirectional BOOST//BUCK - Batt/Discrete PI Controller3 ==
  note: Discrete PID Controller
  note: Pierre Giroux, Gilbert Sybille
      | Power System Simulation Laboratory
      | IREQ, Hydro-Quebc
  Error : Inport  SampleTime=Ts
  Discrete-Time Integrator : DiscreteIntegrator  InitialCondition=Init  SampleTime=Ts  LimitOutput=on  UpperSaturationLimit=UpperLimit  LowerSaturationLimit=LowerLimit  ICPrevOutput=DiscIntNeverNeededParam  ICPrevScaledInput=DiscIntNeverNeededParam
  Kp4 : Gain  Gain=Kp  SaturateOnIntegerOverflow=on  SampleTime=Ts  OutDataTypeStr=Inherit: Same as input  ParamDataTypeStr=Inherit: Same as input
  Kp5 : Gain  Gain=Ki  SaturateOnIntegerOverflow=on  SampleTime=Ts  OutDataTypeStr=Inherit: Same as input  ParamDataTypeStr=Inherit: Same as input
  Saturation2 : Saturate  UpperLimit=UpperLimit  LowerLimit=LowerLimit  SampleTime=Ts
  Sum6 : Sum  InputSameDT=on  SaturateOnIntegerOverflow=on  SampleTime=Ts  OutDataTypeStr=Inherit: Same as first input
  Zero-Order Hold : ZeroOrderHold  SampleTime=Ts
  Out : Outport  SampleTime=Ts  InitialOutput=0  VectorParamsAs1DForOutWhenUnconnected=off
  wires:
  Zero-Order Hold/1 -> Sum6/1
  Saturation2/1 -> Out/1
  Discrete-Time Integrator/1 -> Sum6/2
  Kp4/1 -> Zero-Order Hold/1
  Kp5/1 -> Discrete-Time Integrator/1
  Sum6/1 -> Saturation2/1
  Error/1 -> Kp5/1, Kp4/1

== system lib_converters/Bidirectional BOOST//BUCK - Batt/Discrete PI Controller4 ==
  note: Pierre Giroux, Gilbert Sybille
      | Power System Simulation Laboratory
      | IREQ, Hydro-Quebc
  note: Discrete PID Controller
  Error : Inport  SampleTime=Ts
  Discrete-Time Integrator : DiscreteIntegrator  InitialCondition=Init  SampleTime=Ts  LimitOutput=on  UpperSaturationLimit=UpperLimit  LowerSaturationLimit=LowerLimit  ICPrevOutput=DiscIntNeverNeededParam  ICPrevScaledInput=DiscIntNeverNeededParam
  Kp4 : Gain  Gain=Kp  SaturateOnIntegerOverflow=on  SampleTime=Ts  OutDataTypeStr=Inherit: Same as input  ParamDataTypeStr=Inherit: Same as input
  Kp5 : Gain  Gain=Ki  SaturateOnIntegerOverflow=on  SampleTime=Ts  OutDataTypeStr=Inherit: Same as input  ParamDataTypeStr=Inherit: Same as input
  Saturation2 : Saturate  UpperLimit=UpperLimit  LowerLimit=LowerLimit  SampleTime=Ts
  Sum6 : Sum  InputSameDT=on  SaturateOnIntegerOverflow=on  SampleTime=Ts  OutDataTypeStr=Inherit: Same as first input
  Zero-Order Hold : ZeroOrderHold  SampleTime=Ts
  Out : Outport  SampleTime=Ts  InitialOutput=0  VectorParamsAs1DForOutWhenUnconnected=off
  wires:
  Error/1 -> Kp4/1, Kp5/1
  Sum6/1 -> Saturation2/1
  Kp5/1 -> Discrete-Time Integrator/1
  Kp4/1 -> Zero-Order Hold/1
  Discrete-Time Integrator/1 -> Sum6/2
  Saturation2/1 -> Out/1
  Zero-Order Hold/1 -> Sum6/1

== system lib_converters/Bidirectional BOOST//BUCK - Batt - fast/Discrete PI Controller1 ==
  note: Discrete PID Controller
  note: Pierre Giroux, Gilbert Sybille
      | Power System Simulation Laboratory
      | IREQ, Hydro-Quebc
  Error : Inport  SampleTime=Ts
  Discrete-Time Integrator : DiscreteIntegrator  InitialCondition=Init  SampleTime=Ts  LimitOutput=on  UpperSaturationLimit=UpperLimit  LowerSaturationLimit=LowerLimit  ICPrevOutput=DiscIntNeverNeededParam  ICPrevScaledInput=DiscIntNeverNeededParam
  Kp4 : Gain  Gain=Kp  SaturateOnIntegerOverflow=on  SampleTime=Ts  OutDataTypeStr=Inherit: Same as input  ParamDataTypeStr=Inherit: Same as input
  Kp5 : Gain  Gain=Ki  SaturateOnIntegerOverflow=on  SampleTime=Ts  OutDataTypeStr=Inherit: Same as input  ParamDataTypeStr=Inherit: Same as input
  Saturation2 : Saturate  UpperLimit=UpperLimit  LowerLimit=LowerLimit  SampleTime=Ts
  Sum6 : Sum  InputSameDT=on  SaturateOnIntegerOverflow=on  SampleTime=Ts  OutDataTypeStr=Inherit: Same as first input
  Zero-Order Hold : ZeroOrderHold  SampleTime=Ts
  Out : Outport  SampleTime=Ts  InitialOutput=0  VectorParamsAs1DForOutWhenUnconnected=off
  wires:
  Zero-Order Hold/1 -> Sum6/1
  Saturation2/1 -> Out/1
  Discrete-Time Integrator/1 -> Sum6/2
  Kp4/1 -> Zero-Order Hold/1
  Kp5/1 -> Discrete-Time Integrator/1
  Sum6/1 -> Saturation2/1
  Error/1 -> Kp5/1, Kp4/1

== system lib_converters/Bidirectional BOOST//BUCK - Batt - fast/Discrete PI Controller2 ==
  note: Pierre Giroux, Gilbert Sybille
      | Power System Simulation Laboratory
      | IREQ, Hydro-Quebc
  note: Discrete PID Controller
  Error : Inport  SampleTime=Ts
  Discrete-Time Integrator : DiscreteIntegrator  InitialCondition=Init  SampleTime=Ts  LimitOutput=on  UpperSaturationLimit=UpperLimit  LowerSaturationLimit=LowerLimit  ICPrevOutput=DiscIntNeverNeededParam  ICPrevScaledInput=DiscIntNeverNeededParam
  Kp4 : Gain  Gain=Kp  SaturateOnIntegerOverflow=on  SampleTime=Ts  OutDataTypeStr=Inherit: Same as input  ParamDataTypeStr=Inherit: Same as input
  Kp5 : Gain  Gain=Ki  SaturateOnIntegerOverflow=on  SampleTime=Ts  OutDataTypeStr=Inherit: Same as input  ParamDataTypeStr=Inherit: Same as input
  Saturation2 : Saturate  UpperLimit=UpperLimit  LowerLimit=LowerLimit  SampleTime=Ts
  Sum6 : Sum  InputSameDT=on  SaturateOnIntegerOverflow=on  SampleTime=Ts  OutDataTypeStr=Inherit: Same as first input
  Zero-Order Hold : ZeroOrderHold  SampleTime=Ts
  Out : Outport  SampleTime=Ts  InitialOutput=0  VectorParamsAs1DForOutWhenUnconnected=off
  wires:
  Error/1 -> Kp4/1, Kp5/1
  Sum6/1 -> Saturation2/1
  Kp5/1 -> Discrete-Time Integrator/1
  Kp4/1 -> Zero-Order Hold/1
  Discrete-Time Integrator/1 -> Sum6/2
  Saturation2/1 -> Out/1
  Zero-Order Hold/1 -> Sum6/1

== system lib_converters/Bidirectional BOOST//BUCK - Batt - fast/Discrete PI Controller3 ==
  note: Pierre Giroux, Gilbert Sybille
      | Power System Simulation Laboratory
      | IREQ, Hydro-Quebc
  note: Discrete PID Controller
  Error : Inport  SampleTime=Ts
  Discrete-Time Integrator : DiscreteIntegrator  InitialCondition=Init  SampleTime=Ts  LimitOutput=on  UpperSaturationLimit=UpperLimit  LowerSaturationLimit=LowerLimit  ICPrevOutput=DiscIntNeverNeededParam  ICPrevScaledInput=DiscIntNeverNeededParam
  Kp4 : Gain  Gain=Kp  SaturateOnIntegerOverflow=on  SampleTime=Ts  OutDataTypeStr=Inherit: Same as input  ParamDataTypeStr=Inherit: Same as input
  Kp5 : Gain  Gain=Ki  SaturateOnIntegerOverflow=on  SampleTime=Ts  OutDataTypeStr=Inherit: Same as input  ParamDataTypeStr=Inherit: Same as input
  Saturation2 : Saturate  UpperLimit=UpperLimit  LowerLimit=LowerLimit  SampleTime=Ts
  Sum6 : Sum  InputSameDT=on  SaturateOnIntegerOverflow=on  SampleTime=Ts  OutDataTypeStr=Inherit: Same as first input
  Zero-Order Hold : ZeroOrderHold  SampleTime=Ts
  Out : Outport  SampleTime=Ts  InitialOutput=0  VectorParamsAs1DForOutWhenUnconnected=off
  wires:
  Error/1 -> Kp4/1, Kp5/1
  Sum6/1 -> Saturation2/1
  Kp5/1 -> Discrete-Time Integrator/1
  Kp4/1 -> Zero-Order Hold/1
  Discrete-Time Integrator/1 -> Sum6/2
  Saturation2/1 -> Out/1
  Zero-Order Hold/1 -> Sum6/1

== system lib_converters/Bidirectional BOOST//BUCK - Batt - fast/Discrete PI Controller4 ==
  note: Discrete PID Controller
  note: Pierre Giroux, Gilbert Sybille
      | Power System Simulation Laboratory
      | IREQ, Hydro-Quebc
  Error : Inport  SampleTime=Ts
  Discrete-Time Integrator : DiscreteIntegrator  InitialCondition=Init  SampleTime=Ts  LimitOutput=on  UpperSaturationLimit=UpperLimit  LowerSaturationLimit=LowerLimit  ICPrevOutput=DiscIntNeverNeededParam  ICPrevScaledInput=DiscIntNeverNeededParam
  Kp4 : Gain  Gain=Kp  SaturateOnIntegerOverflow=on  SampleTime=Ts  OutDataTypeStr=Inherit: Same as input  ParamDataTypeStr=Inherit: Same as input
  Kp5 : Gain  Gain=Ki  SaturateOnIntegerOverflow=on  SampleTime=Ts  OutDataTypeStr=Inherit: Same as input  ParamDataTypeStr=Inherit: Same as input
  Saturation2 : Saturate  UpperLimit=UpperLimit  LowerLimit=LowerLimit  SampleTime=Ts
  Sum6 : Sum  InputSameDT=on  SaturateOnIntegerOverflow=on  SampleTime=Ts  OutDataTypeStr=Inherit: Same as first input
  Zero-Order Hold : ZeroOrderHold  SampleTime=Ts
  Out : Outport  SampleTime=Ts  InitialOutput=0  VectorParamsAs1DForOutWhenUnconnected=off
  wires:
  Zero-Order Hold/1 -> Sum6/1
  Saturation2/1 -> Out/1
  Discrete-Time Integrator/1 -> Sum6/2
  Kp4/1 -> Zero-Order Hold/1
  Kp5/1 -> Discrete-Time Integrator/1
  Sum6/1 -> Saturation2/1
  Error/1 -> Kp5/1, Kp4/1

== system lib_converters/Bidirectional BOOST//BUCK - avg-swh/Discrete PI Controller1 ==
  note: Discrete PID Controller
  note: Pierre Giroux, Gilbert Sybille
      | Power System Simulation Laboratory
      | IREQ, Hydro-Quebc
  Error : Inport  SampleTime=Ts
  Discrete-Time Integrator : DiscreteIntegrator  InitialCondition=Init  SampleTime=Ts  LimitOutput=on  UpperSaturationLimit=UpperLimit  LowerSaturationLimit=LowerLimit  ICPrevOutput=DiscIntNeverNeededParam  ICPrevScaledInput=DiscIntNeverNeededParam
  Kp4 : Gain  Gain=Kp  SaturateOnIntegerOverflow=on  SampleTime=Ts  OutDataTypeStr=Inherit: Same as input  ParamDataTypeStr=Inherit: Same as input
  Kp5 : Gain  Gain=Ki  SaturateOnIntegerOverflow=on  SampleTime=Ts  OutDataTypeStr=Inherit: Same as input  ParamDataTypeStr=Inherit: Same as input
  Saturation2 : Saturate  UpperLimit=UpperLimit  LowerLimit=LowerLimit  SampleTime=Ts
  Sum6 : Sum  InputSameDT=on  SaturateOnIntegerOverflow=on  SampleTime=Ts  OutDataTypeStr=Inherit: Same as first input
  Zero-Order Hold : ZeroOrderHold  SampleTime=Ts
  Out : Outport  SampleTime=Ts  InitialOutput=0  VectorParamsAs1DForOutWhenUnconnected=off
  wires:
  Zero-Order Hold/1 -> Sum6/1
  Saturation2/1 -> Out/1
  Discrete-Time Integrator/1 -> Sum6/2
  Kp4/1 -> Zero-Order Hold/1
  Kp5/1 -> Discrete-Time Integrator/1
  Sum6/1 -> Saturation2/1
  Error/1 -> Kp5/1, Kp4/1

== system lib_converters/Bidirectional BOOST//BUCK - avg-swh/Discrete PI Controller2 ==
  note: Pierre Giroux, Gilbert Sybille
      | Power System Simulation Laboratory
      | IREQ, Hydro-Quebc
  note: Discrete PID Controller
  Error : Inport  SampleTime=Ts
  Discrete-Time Integrator : DiscreteIntegrator  InitialCondition=Init  SampleTime=Ts  LimitOutput=on  UpperSaturationLimit=UpperLimit  LowerSaturationLimit=LowerLimit  ICPrevOutput=DiscIntNeverNeededParam  ICPrevScaledInput=DiscIntNeverNeededParam
  Kp4 : Gain  Gain=Kp  SaturateOnIntegerOverflow=on  SampleTime=Ts  OutDataTypeStr=Inherit: Same as input  ParamDataTypeStr=Inherit: Same as input
  Kp5 : Gain  Gain=Ki  SaturateOnIntegerOverflow=on  SampleTime=Ts  OutDataTypeStr=Inherit: Same as input  ParamDataTypeStr=Inherit: Same as input
  Saturation2 : Saturate  UpperLimit=UpperLimit  LowerLimit=LowerLimit  SampleTime=Ts
  Sum6 : Sum  InputSameDT=on  SaturateOnIntegerOverflow=on  SampleTime=Ts  OutDataTypeStr=Inherit: Same as first input
  Zero-Order Hold : ZeroOrderHold  SampleTime=Ts
  Out : Outport  SampleTime=Ts  InitialOutput=0  VectorParamsAs1DForOutWhenUnconnected=off
  wires:
  Error/1 -> Kp4/1, Kp5/1
  Sum6/1 -> Saturation2/1
  Kp5/1 -> Discrete-Time Integrator/1
  Kp4/1 -> Zero-Order Hold/1
  Discrete-Time Integrator/1 -> Sum6/2
  Saturation2/1 -> Out/1
  Zero-Order Hold/1 -> Sum6/1

== system lib_converters/Bidirectional BOOST//BUCK - avg-swh/Discrete PI Controller3 ==
  note: Pierre Giroux, Gilbert Sybille
      | Power System Simulation Laboratory
      | IREQ, Hydro-Quebc
  note: Discrete PID Controller
  Error : Inport  SampleTime=Ts
  Discrete-Time Integrator : DiscreteIntegrator  InitialCondition=Init  SampleTime=Ts  LimitOutput=on  UpperSaturationLimit=UpperLimit  LowerSaturationLimit=LowerLimit  ICPrevOutput=DiscIntNeverNeededParam  ICPrevScaledInput=DiscIntNeverNeededParam
  Kp4 : Gain  Gain=Kp  SaturateOnIntegerOverflow=on  SampleTime=Ts  OutDataTypeStr=Inherit: Same as input  ParamDataTypeStr=Inherit: Same as input
  Kp5 : Gain  Gain=Ki  SaturateOnIntegerOverflow=on  SampleTime=Ts  OutDataTypeStr=Inherit: Same as input  ParamDataTypeStr=Inherit: Same as input
  Saturation2 : Saturate  UpperLimit=UpperLimit  LowerLimit=LowerLimit  SampleTime=Ts
  Sum6 : Sum  InputSameDT=on  SaturateOnIntegerOverflow=on  SampleTime=Ts  OutDataTypeStr=Inherit: Same as first input
  Zero-Order Hold : ZeroOrderHold  SampleTime=Ts
  Out : Outport  SampleTime=Ts  InitialOutput=0  VectorParamsAs1DForOutWhenUnconnected=off
  wires:
  Error/1 -> Kp4/1, Kp5/1
  Sum6/1 -> Saturation2/1
  Kp5/1 -> Discrete-Time Integrator/1
  Kp4/1 -> Zero-Order Hold/1
  Discrete-Time Integrator/1 -> Sum6/2
  Saturation2/1 -> Out/1
  Zero-Order Hold/1 -> Sum6/1

== system lib_converters/Bidirectional BOOST//BUCK - avg-swh/Discrete PI Controller4 ==
  note: Discrete PID Controller
  note: Pierre Giroux, Gilbert Sybille
      | Power System Simulation Laboratory
      | IREQ, Hydro-Quebc
  Error : Inport  SampleTime=Ts
  Discrete-Time Integrator : DiscreteIntegrator  InitialCondition=Init  SampleTime=Ts  LimitOutput=on  UpperSaturationLimit=UpperLimit  LowerSaturationLimit=LowerLimit  ICPrevOutput=DiscIntNeverNeededParam  ICPrevScaledInput=DiscIntNeverNeededParam
  Kp4 : Gain  Gain=Kp  SaturateOnIntegerOverflow=on  SampleTime=Ts  OutDataTypeStr=Inherit: Same as input  ParamDataTypeStr=Inherit: Same as input
  Kp5 : Gain  Gain=Ki  SaturateOnIntegerOverflow=on  SampleTime=Ts  OutDataTypeStr=Inherit: Same as input  ParamDataTypeStr=Inherit: Same as input
  Saturation2 : Saturate  UpperLimit=UpperLimit  LowerLimit=LowerLimit  SampleTime=Ts
  Sum6 : Sum  InputSameDT=on  SaturateOnIntegerOverflow=on  SampleTime=Ts  OutDataTypeStr=Inherit: Same as first input
  Zero-Order Hold : ZeroOrderHold  SampleTime=Ts
  Out : Outport  SampleTime=Ts  InitialOutput=0  VectorParamsAs1DForOutWhenUnconnected=off
  wires:
  Zero-Order Hold/1 -> Sum6/1
  Saturation2/1 -> Out/1
  Discrete-Time Integrator/1 -> Sum6/2
  Kp4/1 -> Zero-Order Hold/1
  Kp5/1 -> Discrete-Time Integrator/1
  Sum6/1 -> Saturation2/1
  Error/1 -> Kp5/1, Kp4/1

== system lib_converters/Bidirectional BOOST//BUCK - avg-swh/Subsystem ==
  g : Inport
  D : Inport  Port=2
  converter : Inport  Port=3
  avg : Subsystem  VariantControl=Choice
  swh : Subsystem  VariantControl=Choice_1
  R+ : PMIOPort  Side=Right
  L+ : PMIOPort  Port=2  Side=Left
  L- : PMIOPort  Port=3  Side=Left
  R- : PMIOPort  Port=4  Side=Right
  Vbatt : Outport
  Ibatt : Outport  Port=2
  IL : Outport  Port=3
  Idcbus : Outport  Port=4
  Vdcbus : Outport  Port=5
